simulink model "circuit"  (R2021a)
settings: Solver=VariableStepAuto  StartTime=0.0  StopTime=10.0  RelTol=1e-3
libraries: fl_lib x34, nesl_utility x4, ee_lib x1
settings Model: Creator=WH  LastModifiedBy=WH

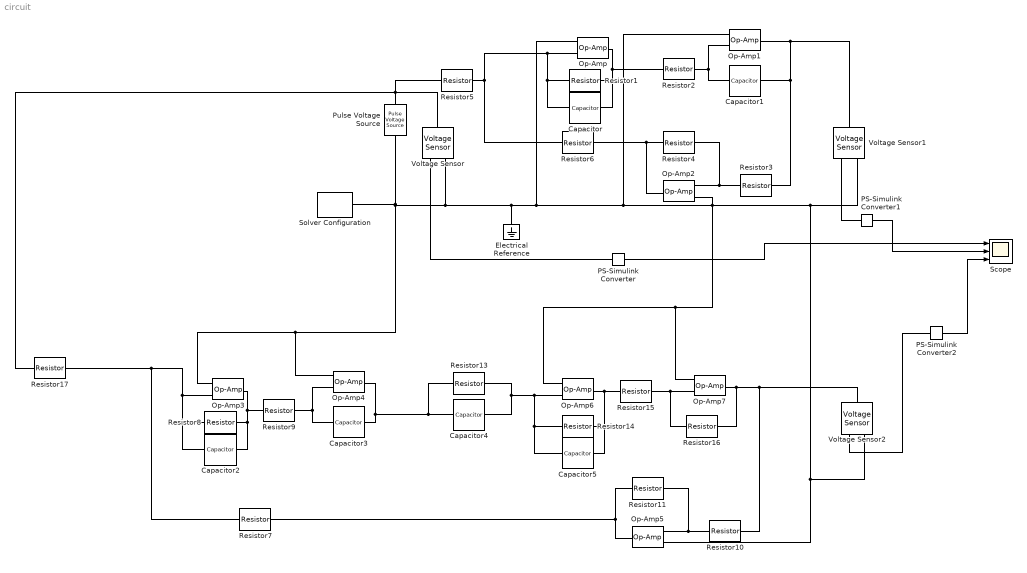
== system circuit ==
  Capacitor{,1..4} (5 alike) : fl_lib/Electrical/Electrical Elements/Capacitor  c=1e-6 F  r=1e-6 Ohm  g=0 1/Ohm  i_specify=off  i_priority=None  i=0 A  i_nominal_specify=off  i_nominal_unit=A  i_nominal_value=1  v_specify=off  v_priority=None  v=0 V  v_nominal_specify=off  v_nominal_unit=V  v_nominal_value=1  vc_specify=off  vc_priority=High  vc=0 V  vc_nominal_specify=off  vc_nominal_unit=V  vc_nominal_value=1
  Capacitor5 : fl_lib/Electrical/Electrical Elements/Capacitor  c=1e-7 F  r=1e-7 Ohm  g=0 1/Ohm  i_specify=off  i_priority=None  i=0 A  i_nominal_specify=off  i_nominal_unit=A  i_nominal_value=1  v_specify=off  v_priority=None  v=0 V  v_nominal_specify=off  v_nominal_unit=V  v_nominal_value=1  vc_specify=off  vc_priority=High  vc=0 V  vc_nominal_specify=off  vc_nominal_unit=V  vc_nominal_value=1
  Electrical Reference : fl_lib/Electrical/Electrical Elements/Electrical Reference
  Op-Amp{,1..7} (8 alike) : fl_lib/Electrical/Electrical Elements/Op-Amp  outI_specify=off  outI_priority=None  outI=0 A  outI_nominal_specify=off  outI_nominal_unit=A  outI_nominal_value=1
  PS-Simulink Converter : nesl_utility/PS-Simulink Converter  PhysicalDomain=network_engine_domain  SubClassName=ps_output  LeftPortType=input  RightPortType=output  PseudoPeriodic=off  Frequencies=[]  Unit=inherit  AffineConversion=off
      settings: SourceProductBaseCode=PW,SS
  PS-Simulink Converter1 : nesl_utility/PS-Simulink Converter  PhysicalDomain=network_engine_domain  SubClassName=ps_output  LeftPortType=input  RightPortType=output  PseudoPeriodic=off  Frequencies=[]  Unit=inherit  AffineConversion=off
      settings: SourceProductBaseCode=PW,SS
  PS-Simulink Converter2 : nesl_utility/PS-Simulink Converter  PhysicalDomain=network_engine_domain  SubClassName=ps_output  LeftPortType=input  RightPortType=output  PseudoPeriodic=off  Frequencies=[]  Unit=inherit  AffineConversion=off
      settings: SourceProductBaseCode=PW,SS
  Pulse Voltage Source : ee_lib/Additional Components/SPICE Sources/Pulse Voltage Source  V1=0 V  V2=1 V  TD=100 ms  TR=1e-9 s  TF=1e-9 s  PW=Inf s  PER=Inf s
      settings: SourceProductBaseCode=PS  InternalSimscapePortConfiguration="{\"Bottom\":[],\"Left\":[{\"id\":\"p\",\"label\":\"\",\"type\":\"foundation.electrical.electrical\"}],\"Right\":[{\"id\":\"n\",\"label\":\"\",\"type\":\"foundation.electrical.electrical\"}],\"Top\":[]}"
  Resistor1 : fl_lib/Electrical/Electrical Elements/Resistor  R=500 kOhm  i_specify=off  i_priority=None  i=0 A  i_nominal_specify=off  i_nominal_unit=A  i_nominal_value=1  v_specify=off  v_priority=None  v=0 V  v_nominal_specify=off  v_nominal_unit=V  v_nominal_value=1
  Resistor{3..7,10..11,15,17} (9 alike) : fl_lib/Electrical/Electrical Elements/Resistor  R=100 kOhm  i_specify=off  i_priority=None  i=0 A  i_nominal_specify=off  i_nominal_unit=A  i_nominal_value=1  v_specify=off  v_priority=None  v=0 V  v_nominal_specify=off  v_nominal_unit=V  v_nominal_value=1
  Resistor13 : fl_lib/Electrical/Electrical Elements/Resistor  R=200 kOhm  i_specify=off  i_priority=None  i=0 A  i_nominal_specify=off  i_nominal_unit=A  i_nominal_value=1  v_specify=off  v_priority=None  v=0 V  v_nominal_specify=off  v_nominal_unit=V  v_nominal_value=1
  Resistor14 : fl_lib/Electrical/Electrical Elements/Resistor  R=400 kOhm  i_specify=off  i_priority=None  i=0 A  i_nominal_specify=off  i_nominal_unit=A  i_nominal_value=1  v_specify=off  v_priority=None  v=0 V  v_nominal_specify=off  v_nominal_unit=V  v_nominal_value=1
  Resistor16 : fl_lib/Electrical/Electrical Elements/Resistor  R=50 kOhm  i_specify=off  i_priority=None  i=0 A  i_nominal_specify=off  i_nominal_unit=A  i_nominal_value=1  v_specify=off  v_priority=None  v=0 V  v_nominal_specify=off  v_nominal_unit=V  v_nominal_value=1
  Resistor2 : fl_lib/Electrical/Electrical Elements/Resistor  R=200 kOhm  i_specify=off  i_priority=None  i=0 A  i_nominal_specify=off  i_nominal_unit=A  i_nominal_value=1  v_specify=off  v_priority=None  v=0 V  v_nominal_specify=off  v_nominal_unit=V  v_nominal_value=1
  Resistor8 : fl_lib/Electrical/Electrical Elements/Resistor  R=500 kOhm  i_specify=off  i_priority=None  i=0 A  i_nominal_specify=off  i_nominal_unit=A  i_nominal_value=1  v_specify=off  v_priority=None  v=0 V  v_nominal_specify=off  v_nominal_unit=V  v_nominal_value=1
  Resistor9 : fl_lib/Electrical/Electrical Elements/Resistor  R=200 kOhm  i_specify=off  i_priority=None  i=0 A  i_nominal_specify=off  i_nominal_unit=A  i_nominal_value=1  v_specify=off  v_priority=None  v=0 V  v_nominal_specify=off  v_nominal_unit=V  v_nominal_value=1
  Scope : Scope  NumInputPorts=3
  Solver Configuration : nesl_utility/Solver Configuration  PhysicalDomain=network_engine_domain  SubClassName=solver  LeftPortType=input  RightPortType=generic  Tones=[]  Harmonics=[]  SimulateNoise=off  Profile=off  UseLocalSampling=off  EnableSwitchedLinearOptims=on  FrequencyDomain=off  UseCCode=off  RelTol=0.001  AbsTol=1e-06  MinStep=1e-09  ToWorkspace=off  RevertToSquareIcSolve=off  NumHomotopyIterations=100  PhasorMode=off  PhasorModeNumHarmonics=1  DoDC=off  ResidualTolerance=1e-09  UseLocalSolver=off  LocalSolverChoice=NE_BACKWARD_EULER_ADVANCER  LocalSolverSampleTime=0.001  DoFixedCost=off  MaxNonlinIter=3  MaxModeIter=2  ComputeImpulses=off  ImpulseIterations=2  LinearAlgebra=auto  EquationFormulation=NE_TIME_EF  DelaysMemoryBudget=1024  AutomaticFiltering=on  FilteringTimeConstant=0.001  PartitionStorageMethod=AS_NEEDED  PartitionMemoryBudget=1024  PartitionMethod=ROBUST
      settings: SourceProductBaseCode=PW,SS
  Voltage Sensor : fl_lib/Electrical/Electrical Sensors/Voltage Sensor
  Voltage Sensor1 : fl_lib/Electrical/Electrical Sensors/Voltage Sensor
  Voltage Sensor2 : fl_lib/Electrical/Electrical Sensors/Voltage Sensor
  wires:
  PS-Simulink Converter/1 -> Scope/1
  PS-Simulink Converter1/1 -> Scope/2
  PS-Simulink Converter2/1 -> Scope/3
  connections:
  Resistor1/RConn1 -- Resistor2/LConn1 -- Op-Amp/RConn1 -- Capacitor/RConn1
  Resistor2/RConn1 -- Capacitor1/LConn1 -- Op-Amp1/LConn2
  Capacitor1/RConn1 -- Resistor3/RConn1 -- Voltage Sensor1/LConn1 -- Op-Amp1/RConn1
  Op-Amp2/LConn2 -- Resistor4/RConn1 -- Resistor3/LConn1
  Capacitor/LConn1 -- Resistor1/LConn1 -- Resistor6/LConn1 -- Resistor5/RConn1 -- Op-Amp/LConn2
  Pulse Voltage Source/LConn1 -- Resistor17/LConn1 -- Voltage Sensor/LConn1 -- Resistor5/LConn1
  Op-Amp6/LConn1 -- Voltage Sensor2/RConn2 -- Op-Amp5/LConn1 -- Voltage Sensor1/RConn2 -- Op-Amp4/LConn1 -- Op-Amp3/LConn1 -- Pulse Voltage Source/RConn1 -- Solver Configuration/RConn1 -- Voltage Sensor/RConn2 -- Electrical Reference/LConn1 -- Op-Amp/LConn1 -- Op-Amp1/LConn1 -- Op-Amp2/LConn1 -- Op-Amp7/LConn1
  Voltage Sensor/RConn1 -- PS-Simulink Converter/LConn1
  Voltage Sensor1/RConn1 -- PS-Simulink Converter1/LConn1
  Resistor4/LConn1 -- Resistor6/RConn1 -- Op-Amp2/RConn1
  Resistor16/RConn1 -- Op-Amp7/RConn1 -- Resistor10/RConn1 -- Voltage Sensor2/LConn1
  Resistor11/LConn1 -- Resistor7/RConn1 -- Op-Amp5/RConn1
  Capacitor3/LConn1 -- Resistor9/RConn1 -- Op-Amp4/LConn2
  Resistor10/LConn1 -- Op-Amp5/LConn2 -- Resistor11/RConn1
  Resistor8/LConn1 -- Resistor7/LConn1 -- Resistor17/RConn1 -- Op-Amp3/LConn2 -- Capacitor2/LConn1
  Capacitor2/RConn1 -- Resistor8/RConn1 -- Resistor9/LConn1 -- Op-Amp3/RConn1
  Voltage Sensor2/RConn1 -- PS-Simulink Converter2/LConn1
  Op-Amp7/LConn2 -- Resistor16/LConn1 -- Resistor15/RConn1
  Capacitor4/RConn1 -- Resistor13/RConn1 -- Capacitor5/LConn1 -- Resistor14/LConn1 -- Op-Amp6/LConn2
  Op-Amp6/RConn1 -- Resistor15/LConn1 -- Capacitor5/RConn1 -- Resistor14/RConn1
  Capacitor4/LConn1 -- Capacitor3/RConn1 -- Op-Amp4/RConn1 -- Resistor13/LConn1
